simulink model "TwoLevelSvpwm"  (R2019a)
settings: Solver=FixedStepDiscrete  StartTime=0.0  StopTime=2  RelTol=1e-3  EnableMultiTasking=on
values from neighbouring files (symbols this model uses):
  fsw = 40e3    (= 40000)    [TwoLevelSvpwm_parameters.m]
  FundamentalFrequency = 50    [TwoLevelSvpwm_parameters.m]
  Ts = 1e-6    (= 1e-06)    [TwoLevelSvpwm_parameters.m]
undefined symbols (not defined in the file or in its folder): phase
libraries: powerlib x21, powerlib_meascontrol x2
settings Model: Creator=hakan  LastModifiedBy=hakan
settings DataIOCC: LimitDataPoints=on  ReturnWorkspaceOutputs=off
settings OptimizationCC: LifeSpan=inf
settings DebuggingCC: AllowSymbolicDim=off  SFUnexpectedBacktrackingDiag=warning  SFNoUnconditionalDefaultTransitionDiag=warning  ArithmeticOperatorsInVariantConditions=warning
settings ModelReferenceCC: PropagateSignalLabelsOutOfModel=off
settings SFSimCC: SimUseLocalCustomCode=off
settings RTWCC: RTWUseLocalCustomCode=off
settings CodeAppCC: StateflowObjectComments=on
settings GRTTargetCC: TargetLangStandard=C89/C90 (ANSI)
settings ConfigComp: CovMetricSettings=dw  CovHtmlReporting=on  CovSaveCumulativeToWorkspaceVar=on  CovSaveSingleToWorkspaceVar=on  CovExternalEMLEnable=off
settings SimscapeCC: SimscapeNormalizeSystem=off

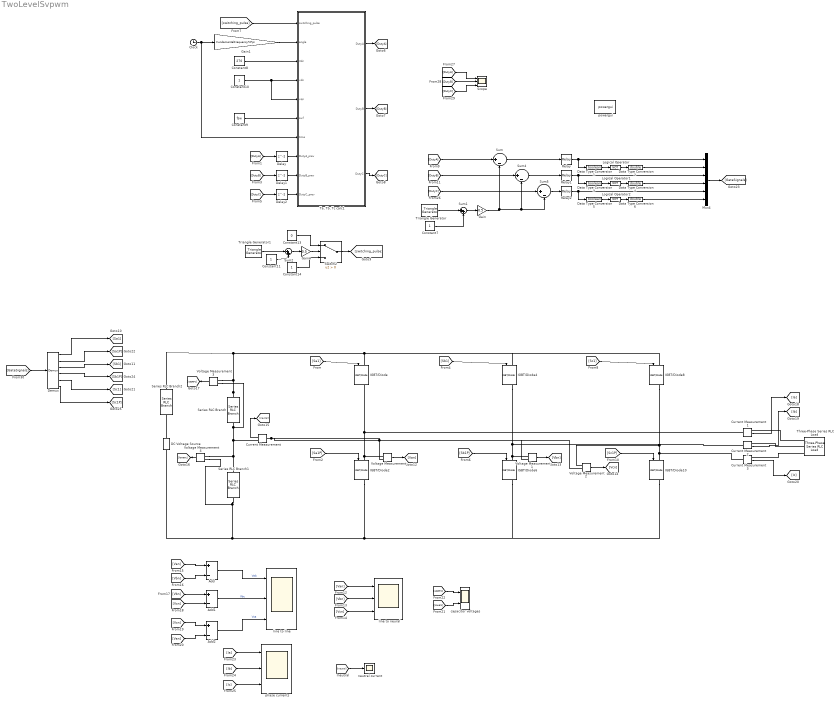
== system TwoLevelSvpwm ==
  Add : Sum  Inputs=+-
  Add1 : Sum  Inputs=+-
  Add2 : Sum  Inputs=+-
  Clock : Clock
  Constant{7,10..11,14} (4 alike) : Constant
  Constant13 : Constant  Value=0
  Constant8 : Constant  Value=270
  Constant9 : Constant  Value=fsw
  Current Measurement{,1..3} (4 alike) : powerlib/Measurements/Current Measurement  PhasorSimulation=off  OutputType=Complex  PSBequivalent=0
      settings: SourceProductName=Simscape Electrical
  DC Voltage Source : powerlib/Electrical Sources/DC Voltage Source  Amplitude=540  Measurements=None
      settings: SourceProductName=Simscape Electrical
  Data Type Conversion1 : DataTypeConversion  OutDataTypeStr=boolean
  Data Type Conversion2 : DataTypeConversion  OutDataTypeStr=double
  Data Type Conversion3 : DataTypeConversion  OutDataTypeStr=boolean
  Data Type Conversion4 : DataTypeConversion  OutDataTypeStr=double
  Data Type Conversion5 : DataTypeConversion  OutDataTypeStr=boolean
  Data Type Conversion6 : DataTypeConversion  OutDataTypeStr=double
  Delay : Delay  DelayLength=1
  Delay1 : Delay  DelayLength=1
  Delay2 : Delay  DelayLength=1
  Demux : Demux  Outputs=6
  Gain : Gain  Gain=0.5
  Gain1 : Gain  Gain=FundamentalFrequency*2*pi
  Gain4 : Gain  Gain=0.5
  IGBT/Diode{,2,4,6,8,10} (6 alike) : powerlib/Power Electronics/IGBT//Diode  Ron=1e-3  Rs=1e5  Cs=inf  Measurements=on
      settings: SourceProductName=Simscape Electrical
  Logical Operator : Logic  Operator=NOT  AllPortsSameDT=off  OutDataTypeStr=boolean
  Logical Operator1 : Logic  Operator=NOT  AllPortsSameDT=off  OutDataTypeStr=boolean
  Logical Operator2 : Logic  Operator=NOT  AllPortsSameDT=off  OutDataTypeStr=boolean
  Mux4 : Mux  Inputs=6
  Relay : Relay
  Relay1 : Relay
  Relay2 : Relay
  Scope : Scope  NumInputPorts=3
  Series RLC Branch : powerlib/Elements/Series RLC Branch  LConnTagsString=__new0  RConnTagsString=__new0  BranchType=C  Resistance=1  Inductance=1e-3  SetiL0=off  InitialCurrent=0  Capacitance=1000e-6  Setx0=off  InitialVoltage=0  Measurements=None
      settings: SourceProductName=Simscape Electrical
  Series RLC Branch1 : powerlib/Elements/Series RLC Branch  LConnTagsString=__new0  RConnTagsString=__new0  BranchType=C  Resistance=1  Inductance=1e-3  SetiL0=off  InitialCurrent=0  Capacitance=1000e-6  Setx0=off  InitialVoltage=0  Measurements=None
      settings: SourceProductName=Simscape Electrical
  Series RLC Branch2 : powerlib/Elements/Series RLC Branch  LConnTagsString=__new0  RConnTagsString=__new0  BranchType=R  Resistance=1  Inductance=1e-3  SetiL0=off  InitialCurrent=0  Capacitance=1000e-6  Setx0=off  InitialVoltage=0  Measurements=None
      settings: SourceProductName=Simscape Electrical
  Sum : Sum  Inputs=|+-
  Sum1 : Sum  Inputs=|++
  Sum2 : Sum  Inputs=|++
  Sum4 : Sum  Inputs=|+-
  Sum5 : Sum  Inputs=|+-
  Switch2 : Switch  Criteria=u2 > Threshold
  "Ta, Tb, Tc calc1" : MATLAB Function  TreatAsAtomicUnit=on
  Three-Phase Series RLC Load : powerlib/Elements/Three-Phase Series RLC Load  LConnTagsString=A|B|C  Configuration=Y (floating)  NominalVoltage=1000  Vabc=[1e3 1e3 1e3]  Vabcp=[1e3 1e3 1e3]  NominalFrequency=50  UnbalancedPower=off  ActivePower=8000  InductivePower=3870  CapacitivePower=0  Pabc=[10e3 9e3 11e3]  QLabc=[100 90 110]  QCabc=[100 90 110]  Pabcp=[10e3 9e3 11e3]  QLabcp=[100 90 110]  QCabcp=[100 90 110]  Measurements=None  LoadType=constant Z
      settings: SourceProductName=Simscape Electrical
  Triangle Generator : powerlib_meascontrol/Pulse & Signal Generators/Triangle Generator  Freq=fsw  Phase=phase(1)  Ts=Ts
      settings: SourceProductName=Simscape Electrical
  Triangle Generator1 : powerlib_meascontrol/Pulse & Signal Generators/Triangle Generator  Freq=fsw  Phase=0  Ts=Ts
      settings: SourceProductName=Simscape Electrical
  Voltage Measurement{,1..4} (5 alike) : powerlib/Measurements/Voltage Measurement  PhasorSimulation=off  OutputType=Complex  PSBequivalent=0
      settings: SourceProductName=Simscape Electrical
  capacitor voltages : Scope  NumInputPorts=2
  line to line : Scope  NumInputPorts=3
  line to neural : Scope  NumInputPorts=3
  neutral current : Scope
  phase currents : Scope  NumInputPorts=3
  powergui : powerlib/powergui  Priority=1  SimulationMode=Discrete  SampleTime=Ts  frequency=60  Iterations=50  frequencyindice=0  Pbase=100e6  ErrMax=1e-4  UnitsV=kV  UnitsW=MW  buscounter=0  FunctionMessages=off  echomessages=off  EnableUseOfTLC=off  CurrentSourceSwitches=off  DisableSnubberDevices=off  DisableRonSwitches=off  DisableVfSwitches=off  DisplayEquations=off  AutomaticDiscreteSolvers=off  SolverType=Tustin/Backward Euler (TBE)  Interpol=off  ExternalGateDelay=off  methode=off  Ts=10  x0status=blocks  SPID=off  SwTol=0  HookPort=off  NonlinearTolerance=0  nMaxIteration=15  ContinueOnMaxIteration=off  RestoreLinks=warning  ResistiveCurrentMeasurement=off  Frange=[0:2:500]  Ylog=off  Xlog=on  ShowGrid=off  save=off  variable=ZData  structure=linetoline  ZoomFFT=off  StartTime=0.0  cycles=2  DisplayStyle=1  fundamental=50  FreqAxis=off  MaxFrequency=5000  frequencyindicesteady=1  RmsSteady=1  display=off
      settings: SourceProductName=Simscape Electrical
  wires:
  [Ineutral] -> neutral current/1
  [Ib] -> phase currents/2
  [Ia] -> phase currents/1
  [Ic] -> phase currents/3
  [Van] -> Add/1
  [Vbn] -> Add/2
  Add/1 -> line to line/1  "Vab"
  [Vbn] -> Add1/1
  [Vcn] -> Add1/2
  Add1/1 -> line to line/2  "Vbc"
  [Vcn] -> Add2/1
  [Van] -> Add2/2
  Add2/1 -> line to line/3  "Vca"
  [Van] -> line to neural/1
  [Vbn] -> line to neural/2
  [Vcn] -> line to neural/3
  [lowerc] -> capacitor voltages/2
  [upperc] -> capacitor voltages/1
  [Sa1] -> IGBT/Diode/1
  [Sa1P] -> IGBT/Diode2/1
  [Sb1] -> IGBT/Diode4/1
  [Sb1P] -> IGBT/Diode6/1
  [Sc1] -> IGBT/Diode8/1
  [Sc1P] -> IGBT/Diode10/1
  Voltage Measurement/1 -> [Van]
  Voltage Measurement1/1 -> [Vbn]
  Voltage Measurement2/1 -> [Vcn]
  Voltage Measurement3/1 -> [upperc]
  Voltage Measurement4/1 -> [lowerc]
  Current Measurement/1 -> [Ineutral]
  Current Measurement1/1 -> [Ia]
  Current Measurement2/1 -> [Ib]
  Current Measurement3/1 -> [Ic]
  Logical Operator1/1 -> Data Type Conversion4/1
  Data Type Conversion6/1 -> Mux4/6
  Relay/1 -> Mux4/1, Data Type Conversion1/1
  Logical Operator/1 -> Data Type Conversion2/1
  Relay1/1 -> Data Type Conversion3/1, Mux4/3
  Data Type Conversion1/1 -> Logical Operator/1
  Sum/1 -> Relay/1
  Triangle Generator/1 -> Sum1/1
  Data Type Conversion3/1 -> Logical Operator1/1
  Data Type Conversion4/1 -> Mux4/4
  [DutyB] -> Sum4/1
  Mux4/1 -> [GateSignals]
  Logical Operator2/1 -> Data Type Conversion6/1
  Data Type Conversion5/1 -> Logical Operator2/1
  Data Type Conversion2/1 -> Mux4/2
  Sum4/1 -> Relay1/1
  Sum5/1 -> Relay2/1
  Relay2/1 -> Data Type Conversion5/1, Mux4/5
  [DutyC] -> Sum5/1
  [DutyA] -> Sum/1
  Sum1/1 -> Gain/1
  Constant7/1 -> Sum1/2
  Gain/1 -> Sum5/2, Sum4/2, Sum/2
  Gain1/1 -> "Ta, Tb, Tc calc1"/2(angle)
  Clock/1 -> "Ta, Tb, Tc calc1"/7(time), Gain1/1
  Constant8/1 -> "Ta, Tb, Tc calc1"/3(Vdc)
  Constant9/1 -> "Ta, Tb, Tc calc1"/6(swf)
  Constant10/1 -> "Ta, Tb, Tc calc1"/5(vqs), "Ta, Tb, Tc calc1"/4(vds)
  "Ta, Tb, Tc calc1"/1(DutyA) -> [DutyA]
  "Ta, Tb, Tc calc1"/2(DutyB) -> [DutyB]
  "Ta, Tb, Tc calc1"/3(DutyC) -> [DutyC]
  [DutyC] -> Delay2/1
  [DutyB] -> Delay1/1
  [DutyA] -> Delay/1
  Delay/1 -> "Ta, Tb, Tc calc1"/8(DutyA_prev)
  Delay1/1 -> "Ta, Tb, Tc calc1"/9(DutyB_prev)
  Delay2/1 -> "Ta, Tb, Tc calc1"/10(DutyC_prev)
  Gain4/1 -> Switch2/2
  Constant13/1 -> Switch2/1
  Switch2/1 -> [switching_pulse]
  Constant11/1 -> Sum2/2
  Constant14/1 -> Switch2/3
  Triangle Generator1/1 -> Sum2/1
  Sum2/1 -> Gain4/1
  [switching_pulse] -> "Ta, Tb, Tc calc1"/1(switching_pulse)
  [DutyB] -> Scope/2
  [DutyA] -> Scope/1
  [DutyC] -> Scope/3
  [GateSignals] -> Demux/1
  Demux/1 -> [Sa1]
  Demux/2 -> [Sa1P]
  Demux/3 -> [Sb1]
  Demux/4 -> [Sb1P]
  Demux/5 -> [Sc1]
  Demux/6 -> [Sc1P]
  connections:
  Series RLC Branch/LConn1 -- Voltage Measurement3/LConn1 -- Series RLC Branch2/LConn1 -- IGBT/Diode/LConn1 -- IGBT/Diode4/LConn1 -- IGBT/Diode8/LConn1
  Voltage Measurement4/LConn2 -- Series RLC Branch1/RConn1 -- DC Voltage Source/LConn1 -- IGBT/Diode2/RConn1 -- IGBT/Diode10/RConn1 -- IGBT/Diode6/RConn1
  Current Measurement1/LConn1 -- IGBT/Diode/RConn1 -- IGBT/Diode2/LConn1 -- Voltage Measurement/LConn1
  Current Measurement/LConn1 -- Voltage Measurement/LConn2 -- Voltage Measurement2/LConn2 -- Voltage Measurement1/LConn2
  Current Measurement2/LConn1 -- IGBT/Diode4/RConn1 -- IGBT/Diode6/LConn1 -- Voltage Measurement1/LConn1
  Voltage Measurement2/LConn1 -- IGBT/Diode10/LConn1 -- Current Measurement3/LConn1 -- IGBT/Diode8/RConn1
  Voltage Measurement3/LConn2 -- Series RLC Branch/RConn1 -- Current Measurement/RConn1 -- Series RLC Branch1/LConn1 -- Voltage Measurement4/LConn1
  Three-Phase Series RLC Load/LConn3 -- Current Measurement3/RConn1
  Three-Phase Series RLC Load/LConn1 -- Current Measurement1/RConn1
  Three-Phase Series RLC Load/LConn2 -- Current Measurement2/RConn1
  DC Voltage Source/RConn1 -- Series RLC Branch2/RConn1

== matlab function TwoLevelSvpwm/Ta, Tb, Tc calc1 ==
  data: switching_pulse input; angle input; Vdc input; vds input; vqs input; swf input; time input; DutyA output; DutyB output; DutyC output; DutyA_prev input; DutyB_prev input; DutyC_prev input
function [DutyA, DutyB, DutyC] = fcn(switching_pulse,angle,Vdc,vds,vqs, swf, time,DutyA_prev, DutyB_prev, DutyC_prev)

Tsw = 1/swf;
T1 = 0;
T2 = 0;
T0 = 0;

% ma = sqrt(vds^2+vqs^2);
% angle = arctan(vqs/vds); % this is an alternative method for getting the

DutyA = 0;
DutyB = 0;
DutyC = 0;

ma = 0.5;
sectornumber = 0;

anglealfa = mod(angle,pi/3);
% T1 = Tsw*ma*sin(pi/3-anglealfa)/(sin(pi/3));
% T2 = Tsw*ma*sin(anglealfa)/(sin(pi/3));
T1 = Tsw*ma*sin(pi/3-anglealfa);
T2 = Tsw*ma*sin(anglealfa);
T0 = Tsw-T1-T2;
if(switching_pulse==1)
    if (mod(angle, 2*pi)<=pi/3)&&(mod(angle, 2*pi)>=0)  % sector 1
        DutyA = (T1+T2+T0/2)/Tsw;
        DutyB = (T2+T0/2)/Tsw;
        DutyC = (T0/2)/Tsw;
        sectornumber = 1;
        return;
    end
    if (mod(angle, 2*pi)<=2*pi/3)&&(mod(angle, 2*pi)>=pi/3)  % sector 2
        DutyA = (T1+T0/2)/Tsw;
        DutyB = (T1+T2+T0/2)/Tsw;
        DutyC = (T0/2)/Tsw;
        sectornumber = 2;
        return;
    end
    if (mod(angle, 2*pi)<=pi)&&(mod(angle, 2*pi)>=2*pi/3)  % sector 3
        if(mod(angle, pi)==0)
        DutyA = (T0/2)/Tsw;
        DutyB = (T1+T0/2)/Tsw;
        DutyC = (T1+T2+T0/2)/Tsw;            
        else
        
        DutyA = (T0/2)/Tsw;
        DutyB = (T1+T2+T0/2)/Tsw;
        DutyC = (T2+T0/2)/Tsw;
        end
        sectornumber = 3;
        return;
    end
    if (mod(angle, 2*pi)<=4*pi/3)&&(mod(angle, 2*pi)>=pi)  % sector 4
        DutyA = (T0/2)/Tsw;
        DutyB = (T1+T0/2)/Tsw;
        DutyC = (T1+T2+T0/2)/Tsw;
        sectornumber = 4;
        return;
    end
    if (mod(angle, 2*pi)<=5*pi/3)&&(mod(angle, 2*pi)>=4*pi/3)  % sector 5
        DutyA = (T2+T0/2)/Tsw;
        DutyB = (T0/2)/Tsw;
        DutyC = (T1+T2+T0/2)/Tsw;
        sectornumber = 5;
        return;
    end
    if (mod(angle, 2*pi)<=2*pi)&&(mod(angle, 2*pi)>=5*pi/3)  % sector 6
        DutyA = (T1+T2+T0/2)/Tsw;
        DutyB = (T0/2)/Tsw;
        DutyC = (T1+T0/2)/Tsw;
        sectornumber = 6;
        return;
    end
else
        DutyA = DutyA_prev;
        DutyB = DutyB_prev;
        DutyC = DutyC_prev;    
end
